simulink model "model_od_transmitancji_podlaczenie"  (R2014b)
settings: Solver=ode45  StartTime=0.0  StopTime=500  RelTol=1e-3
undefined symbols (not defined in the file or in its folder): a1, a2, a3, a4, K, T1, T2, Tp, U, x0
settings Model: Creator=Konrad  LastModifiedBy=Konrad

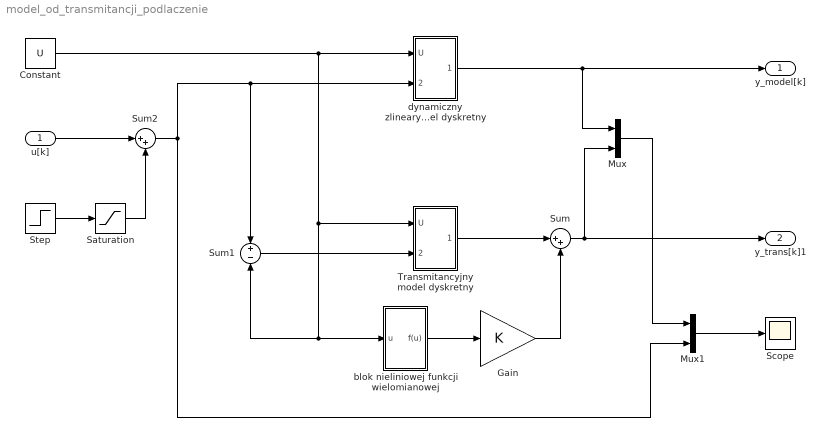
== system model_od_transmitancji_podlaczenie ==
  u[k] : Inport
  Constant : Constant  Value=U
  Gain : Gain  Gain=K
  Mux : Mux  Inputs=2
  Mux1 : Mux  Inputs=2
  Saturation : Saturate  UpperLimit=1  LowerLimit=-1
  Scope : Scope
      settings: YMin=0  YMax=7
  Step : Step  Time=250  After=U  SampleTime=0
  Sum : Sum  Inputs=|++
  Sum1 : Sum  Inputs=+|-
  Sum2 : Sum  Inputs=|++
  Transmitancyjny model dyskretny : Subsystem
  blok nieliniowej funkcji wielomianowej : Subsystem
  dynamiczny zlinearyzowany model dyskretny : Subsystem
  y_model[k] : Outport
  y_trans[k]1 : Outport  Port=2
  wires:
  Step/1 -> Saturation/1
  Mux1/1 -> Scope/1
  Mux/1 -> Mux1/1
  Sum2/1 -> Mux1/2, Sum1/1, dynamiczny zlinearyzowany model dyskretny/2(u[k])
  Constant/1 -> Sum1/2, blok nieliniowej funkcji wielomianowej/1(u), Transmitancyjny model dyskretny/1(U), dynamiczny zlinearyzowany model dyskretny/1(U)
  dynamiczny zlinearyzowany model dyskretny/1(y[k]) -> y_model[k]/1, Mux/1
  Sum1/1 -> Transmitancyjny model dyskretny/2(u[k])
  Transmitancyjny model dyskretny/1(y[k]) -> Sum/1
  Sum/1 -> y_trans[k]1/1, Mux/2
  blok nieliniowej funkcji wielomianowej/1(f(u)) -> Gain/1
  Gain/1 -> Sum/2
  Saturation/1 -> Sum2/2
  u[k]/1 -> Sum2/1

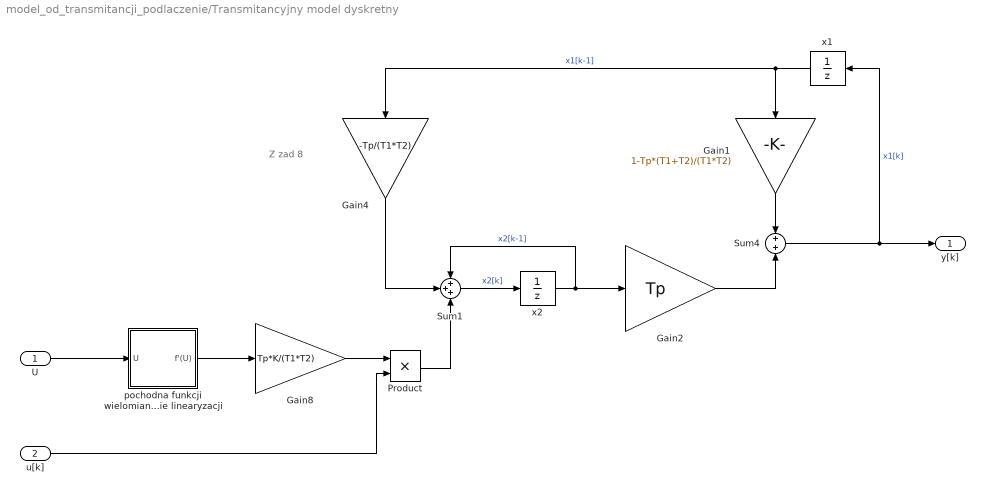
== system model_od_transmitancji_podlaczenie/Transmitancyjny model dyskretny ==
  note: Z zad 8
  U : Inport
  u[k] : Inport  Port=2
  Gain1 : Gain  Gain=1-Tp*(T1+T2)/(T1*T2)
  Gain2 : Gain  Gain=Tp
  Gain4 : Gain  Gain=-Tp/(T1*T2)
  Gain8 : Gain  Gain=Tp*K/(T1*T2)
  Product : Product
  Sum1 : Sum  Inputs=+++
  Sum4 : Sum  Inputs=+|+
  pochodna funkcji wielomianowej w punkcie linearyzacji : Subsystem
  x1 : UnitDelay  InitialCondition=x0(1)  SampleTime=Tp
  x2 : UnitDelay  InitialCondition=x0(2)  SampleTime=Tp
  y[k] : Outport
  wires:
  u[k]/1 -> Product/2
  pochodna funkcji wielomianowej w punkcie linearyzacji/1(f'(U)) -> Gain8/1
  Sum4/1 -> x1/1, y[k]/1  "x1[k]"
  Gain4/1 -> Sum1/2
  x1/1 -> Gain1/1, Gain4/1  "x1[k-1]"
  Gain2/1 -> Sum4/2
  U/1 -> pochodna funkcji wielomianowej w punkcie linearyzacji/1(U)
  Gain1/1 -> Sum4/1
  Sum1/1 -> x2/1  "x2[k]"
  x2/1 -> Gain2/1, Sum1/1  "x2[k-1]"
  Gain8/1 -> Product/1
  Product/1 -> Sum1/3

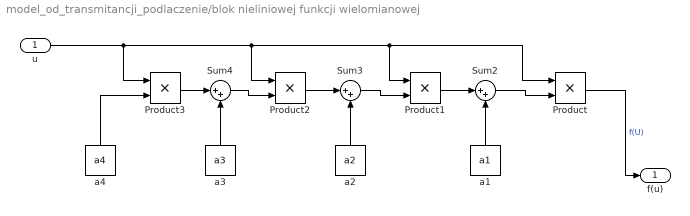
== system model_od_transmitancji_podlaczenie/blok nieliniowej funkcji wielomianowej ==
  u : Inport
  Product{,1..3} (4 alike) : Product
  Sum2 : Sum  Inputs=|++
  Sum3 : Sum  Inputs=|++
  Sum4 : Sum  Inputs=|++
  a1 : Constant  Value=a1
  a2 : Constant  Value=a2
  a3 : Constant  Value=a3
  a4 : Constant  Value=a4
  f(u) : Outport
  wires:
  u/1 -> Product/1, Product1/1, Product2/1, Product3/1
  Product2/1 -> Sum3/1
  Sum2/1 -> Product/2
  Product/1 -> f(u)/1  "f(U)"
  Product3/1 -> Sum4/1
  a1/1 -> Sum2/2
  a2/1 -> Sum3/2
  Sum3/1 -> Product1/2
  Sum4/1 -> Product2/2
  a3/1 -> Sum4/2
  a4/1 -> Product3/2
  Product1/1 -> Sum2/1

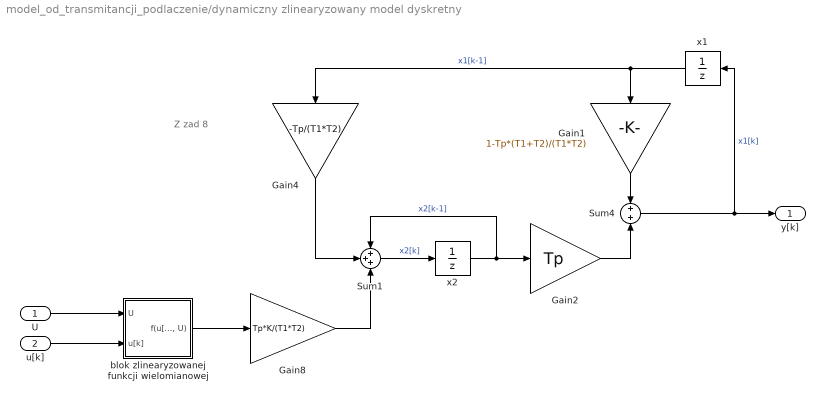
== system model_od_transmitancji_podlaczenie/dynamiczny zlinearyzowany model dyskretny ==
  note: Z zad 8
  U : Inport
  u[k] : Inport  Port=2
  Gain1 : Gain  Gain=1-Tp*(T1+T2)/(T1*T2)
  Gain2 : Gain  Gain=Tp
  Gain4 : Gain  Gain=-Tp/(T1*T2)
  Gain8 : Gain  Gain=Tp*K/(T1*T2)
  Sum1 : Sum  Inputs=+++
  Sum4 : Sum  Inputs=+|+
  blok zlinearyzowanej funkcji wielomianowej : Subsystem
  x1 : UnitDelay  InitialCondition=x0(1)  SampleTime=Tp
  x2 : UnitDelay  InitialCondition=x0(2)  SampleTime=Tp
  y[k] : Outport
  wires:
  u[k]/1 -> blok zlinearyzowanej funkcji wielomianowej/2(u[k])
  blok zlinearyzowanej funkcji wielomianowej/1("f(u[k], U)") -> Gain8/1
  Sum4/1 -> x1/1, y[k]/1  "x1[k]"
  Gain4/1 -> Sum1/2
  x1/1 -> Gain1/1, Gain4/1  "x1[k-1]"
  Gain2/1 -> Sum4/2
  Gain8/1 -> Sum1/3
  U/1 -> blok zlinearyzowanej funkcji wielomianowej/1(U)
  Gain1/1 -> Sum4/1
  Sum1/1 -> x2/1  "x2[k]"
  x2/1 -> Gain2/1, Sum1/1  "x2[k-1]"

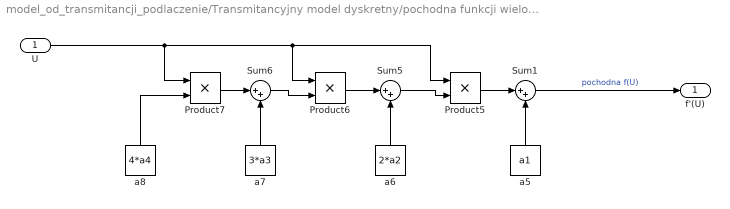
== system model_od_transmitancji_podlaczenie/Transmitancyjny model dyskretny/pochodna funkcji wielomianowej w punkcie linearyzacji ==
  U : Inport
  Product5 : Product
  Product6 : Product
  Product7 : Product
  Sum1 : Sum  Inputs=|++
  Sum5 : Sum  Inputs=|++
  Sum6 : Sum  Inputs=|++
  a5 : Constant  Value=a1
  a6 : Constant  Value=2*a2
  a7 : Constant  Value=3*a3
  a8 : Constant  Value=4*a4
  f'(U) : Outport
  wires:
  U/1 -> Product5/1, Product6/1, Product7/1
  Product5/1 -> Sum1/1
  Product6/1 -> Sum5/1
  Product7/1 -> Sum6/1
  a5/1 -> Sum1/2
  a6/1 -> Sum5/2
  Sum5/1 -> Product5/2
  a7/1 -> Sum6/2
  Sum6/1 -> Product6/2
  a8/1 -> Product7/2
  Sum1/1 -> f'(U)/1  "pochodna f(U)"

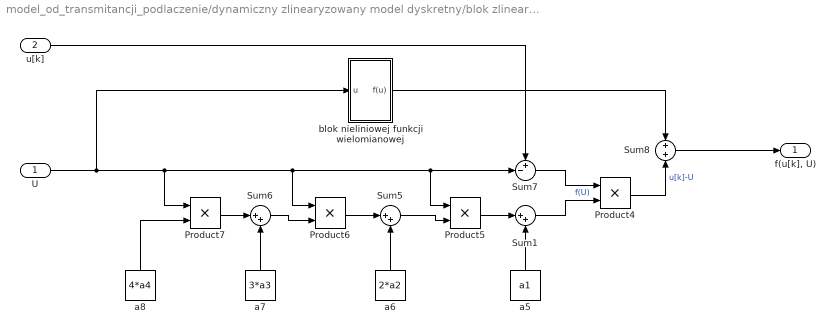
== system model_od_transmitancji_podlaczenie/dynamiczny zlinearyzowany model dyskretny/blok zlinearyzowanej funkcji wielomianowej ==
  U : Inport
  u[k] : Inport  Port=2
  Product{4..7} (4 alike) : Product
  Sum1 : Sum  Inputs=|++
  Sum5 : Sum  Inputs=|++
  Sum6 : Sum  Inputs=|++
  Sum7 : Sum  Inputs=+-|
  Sum8 : Sum
  a5 : Constant  Value=a1
  a6 : Constant  Value=2*a2
  a7 : Constant  Value=3*a3
  a8 : Constant  Value=4*a4
  blok nieliniowej funkcji wielomianowej : Subsystem
  "f(u[k], U)" : Outport
  wires:
  U/1 -> blok nieliniowej funkcji wielomianowej/1(u), Product5/1, Sum7/2, Product6/1, Product7/1
  Product5/1 -> Sum1/1
  Product6/1 -> Sum5/1
  Product7/1 -> Sum6/1
  a5/1 -> Sum1/2
  a6/1 -> Sum5/2
  Sum5/1 -> Product5/2
  a7/1 -> Sum6/2
  Sum6/1 -> Product6/2
  a8/1 -> Product7/2
  Sum1/1 -> Product4/2  "f(U)"
  Sum7/1 -> Product4/1
  u[k]/1 -> Sum7/1
  Product4/1 -> Sum8/2  "u[k]-U"
  Sum8/1 -> "f(u[k], U)"/1
  blok nieliniowej funkcji wielomianowej/1(f(u)) -> Sum8/1

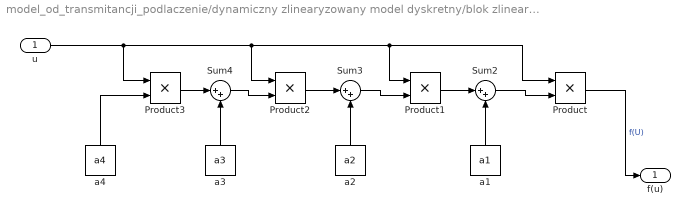
== system model_od_transmitancji_podlaczenie/dynamiczny zlinearyzowany model dyskretny/blok zlinearyzowanej funkcji wielomianowej/blok nieliniowej funkcji wielomianowej ==
  u : Inport
  Product{,1..3} (4 alike) : Product
  Sum2 : Sum  Inputs=|++
  Sum3 : Sum  Inputs=|++
  Sum4 : Sum  Inputs=|++
  a1 : Constant  Value=a1
  a2 : Constant  Value=a2
  a3 : Constant  Value=a3
  a4 : Constant  Value=a4
  f(u) : Outport
  wires:
  u/1 -> Product/1, Product1/1, Product2/1, Product3/1
  Product2/1 -> Sum3/1
  Sum2/1 -> Product/2
  Product/1 -> f(u)/1  "f(U)"
  Product3/1 -> Sum4/1
  a1/1 -> Sum2/2
  a2/1 -> Sum3/2
  Sum3/1 -> Product1/2
  Sum4/1 -> Product2/2
  a3/1 -> Sum4/2
  a4/1 -> Product3/2
  Product1/1 -> Sum2/1
